simulink model "FL"  (R2017a)
settings: Solver=FixedStepAuto  StartTime=0.0  StopTime=100  FixedStep=0.1  RelTol=1e-3
model workspace: external: MAT-File C:\Users\calvinv\Google Drive\code\Matlab\QuadSim\Simulink\cross_section_model\parameters\param.mat (data not in the file)
settings Model: Creator=calvin  LastModifiedBy=calvinv

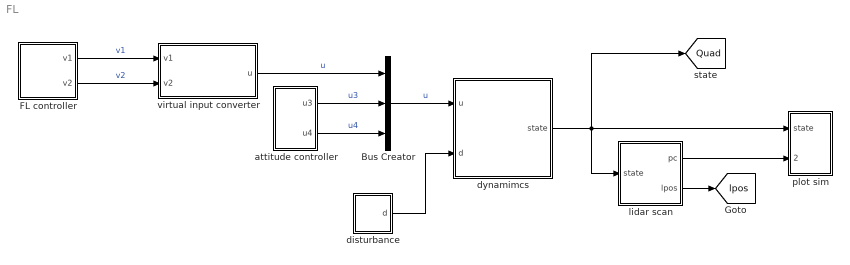
== system FL ==
  Bus Creator : BusCreator  Inputs=3
  FL controller : Subsystem  mask{ky1=10, ky2=42.5, ky3=40.3, ky4=13.4, kz1=10, kz2=42.5, kz3=40.3, kz4=13.4, yd=1, zd=2.5, use_lpos=0}
      mask prompts: yd "target y"; zd "target z"; use_lpos "Use lidar pos feedback"
      mask DialogControl DescGroupVar Prompt: Controller parameters
  attitude controller : Subsystem  mask{P_the=1, D_the=1.5, P_psi=1, D_psi=1.5}
      mask prompts: P_the "Theta P gain"; D_the "Theta D gain"; P_psi "Psi P gain"; D_psi "Pis D gain"
      mask DialogControl DescGroupVar Prompt: Attitude PD controller
  disturbance : Subsystem  mask{freq=20, amp1=0, amp_f=0, amp_tau=0, amp_tau_freq=0, tau_freq=5}
      mask prompts: freq "force oscillation freq"; amp1 "Force amplitude"; amp_f "force oscillation amplitude"; amp_tau "Torque disturbance amplitude"; amp_tau_freq "Torque oscillation freq amp"; tau_freq "Torque oscillation freq"
      mask DialogControl DescGroupVar Prompt: Disturbance generator
  dynamimcs : Subsystem
  lidar scan : Subsystem
  plot sim : Subsystem
  virtual input converter : Subsystem
  tag scope: Quad=global, lpos=global
  wires:
  dynamimcs/1(state) -> lidar scan/1(state), plot sim/1(state), [Quad]
  FL controller/2(v2) -> virtual input converter/2(v2)  "v2"
  FL controller/1(v1) -> virtual input converter/1(v1)  "v1"
  lidar scan/1(pc) -> plot sim/2(lidar pc)
  lidar scan/2(lpos) -> [lpos]
  Bus Creator/1 -> dynamimcs/1(u)  "u"
  attitude controller/1(u3) -> Bus Creator/2  "u3"
  attitude controller/2("u4 ") -> Bus Creator/3  "u4"
  virtual input converter/1(u) -> Bus Creator/1  "u"
  disturbance/1(d) -> dynamimcs/2(d)

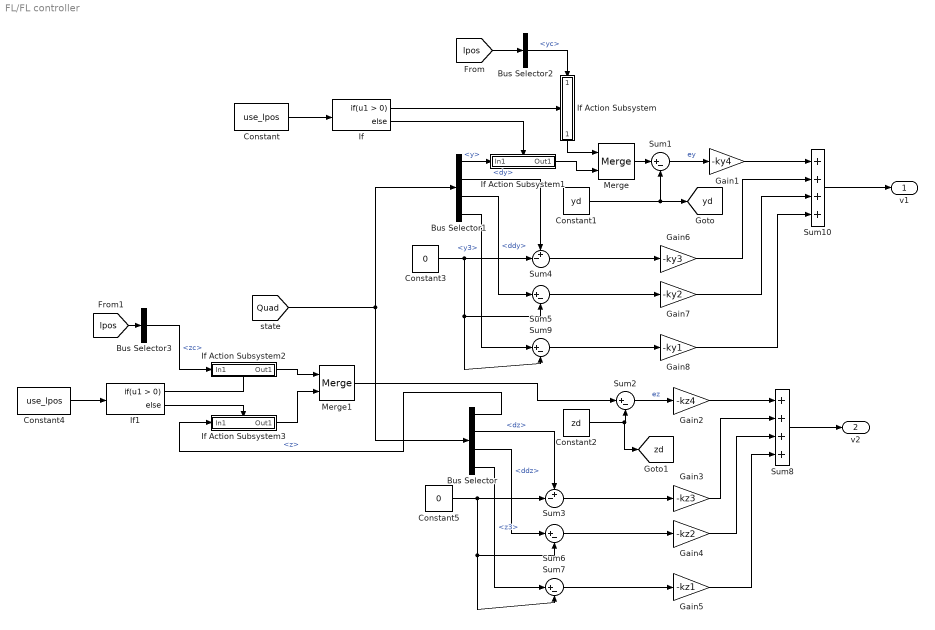
== system FL/FL controller ==
  Bus Selector : BusSelector  OutputSignals=z,dz,ddz,z3
  Bus Selector1 : BusSelector  OutputSignals=y,dy,ddy,y3
  Bus Selector2 : BusSelector  OutputSignals=yc
  Bus Selector3 : BusSelector  OutputSignals=zc
  Constant : Constant  Value=use_lpos
  Constant1 : Constant  Value=yd
  Constant2 : Constant  Value=zd
  Constant3 : Constant  Value=0
  Constant4 : Constant  Value=use_lpos
  Constant5 : Constant  Value=0
  Gain1 : Gain  Gain=-ky4
  Gain2 : Gain  Gain=-kz4
  Gain3 : Gain  Gain=-kz3
  Gain4 : Gain  Gain=-kz2
  Gain5 : Gain  Gain=-kz1
  Gain6 : Gain  Gain=-ky3
  Gain7 : Gain  Gain=-ky2
  Gain8 : Gain  Gain=-ky1
  If : If
  If Action Subsystem : Subsystem  TreatAsAtomicUnit=on
  If Action Subsystem1 : Subsystem  TreatAsAtomicUnit=on
  If Action Subsystem2 : Subsystem  TreatAsAtomicUnit=on
  If Action Subsystem3 : Subsystem  TreatAsAtomicUnit=on
  If1 : If
  Merge : Merge
  Merge1 : Merge
  Sum{1..2,5..7,9} (6 alike) : Sum  Inputs=|+-
  Sum10 : Sum  Inputs=++++
  Sum3 : Sum  Inputs=+-|
  Sum4 : Sum  Inputs=+-|
  Sum8 : Sum  Inputs=++++
  v1 : Outport
  v2 : Outport  Port=2
  tag scope: yd=global, zd=global
  wires:
  Constant5/1 -> Sum7/2, Sum6/2, Sum3/2
  [Quad] -> Bus Selector1/1, Bus Selector/1
  Sum2/1 -> Gain2/1  "ez"
  Constant2/1 -> [zd], Sum2/2
  Bus Selector/2 -> Sum3/1  "<dz>"
  Sum3/1 -> Gain3/1
  Bus Selector/3 -> Sum6/1  "<ddz>"
  Bus Selector/4 -> Sum7/1  "<z3>"
  Sum7/1 -> Gain5/1
  Sum6/1 -> Gain4/1
  Gain2/1 -> Sum8/1
  Sum8/1 -> v2/1
  Gain3/1 -> Sum8/2
  Gain4/1 -> Sum8/3
  Gain5/1 -> Sum8/4
  Gain8/1 -> Sum10/4
  Gain7/1 -> Sum10/3
  Gain6/1 -> Sum10/2
  Sum10/1 -> v1/1
  Gain1/1 -> Sum10/1
  Sum5/1 -> Gain7/1
  Sum9/1 -> Gain8/1
  Bus Selector1/4 -> Sum9/1  "<y3>"
  Bus Selector1/3 -> Sum5/1  "<ddy>"
  Sum4/1 -> Gain6/1
  Bus Selector1/2 -> Sum4/1  "<dy>"
  Constant1/1 -> Sum1/2, [yd]
  Sum1/1 -> Gain1/1  "ey"
  Constant3/1 -> Sum4/2, Sum5/2, Sum9/2
  [lpos] -> Bus Selector2/1
  [lpos] -> Bus Selector3/1
  If/1 -> If Action Subsystem/Action
  If/2 -> If Action Subsystem1/Action
  Bus Selector1/1 -> If Action Subsystem1/1(In1)  "<y>"
  Merge/1 -> Sum1/1
  If Action Subsystem1/1(Out1) -> Merge/2
  If Action Subsystem/1(Out1) -> Merge/1
  Bus Selector2/1 -> If Action Subsystem/1(In1)  "<yc>"
  Constant/1 -> If/1
  If Action Subsystem2/1(Out1) -> Merge1/1
  If Action Subsystem3/1(Out1) -> Merge1/2
  Merge1/1 -> Sum2/1
  If1/1 -> If Action Subsystem2/Action
  If1/2 -> If Action Subsystem3/Action
  Bus Selector3/1 -> If Action Subsystem2/1(In1)  "<zc>"
  Constant4/1 -> If1/1
  Bus Selector/1 -> If Action Subsystem3/1(In1)  "<z>"

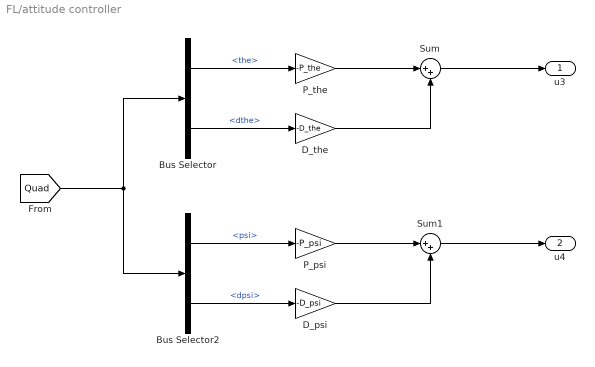
== system FL/attitude controller ==
  Bus Selector : BusSelector  OutputSignals=the,dthe
  Bus Selector2 : BusSelector  OutputSignals=psi,dpsi
  D_psi : Gain  Gain=-D_psi
  D_the : Gain  Gain=-D_the
  P_psi : Gain  Gain=-P_psi
  P_the : Gain  Gain=-P_the
  Sum : Sum  Inputs=|++
  Sum1 : Sum  Inputs=|++
  u3 : Outport
  "u4 " : Outport  Port=2
  wires:
  [Quad] -> Bus Selector2/1, Bus Selector/1
  D_the/1 -> Sum/2
  P_the/1 -> Sum/1
  Bus Selector/2 -> D_the/1  "<dthe>"
  Bus Selector/1 -> P_the/1  "<the>"
  Sum/1 -> u3/1
  Bus Selector2/1 -> P_psi/1  "<psi>"
  Bus Selector2/2 -> D_psi/1  "<dpsi>"
  P_psi/1 -> Sum1/1
  D_psi/1 -> Sum1/2
  Sum1/1 -> "u4 "/1

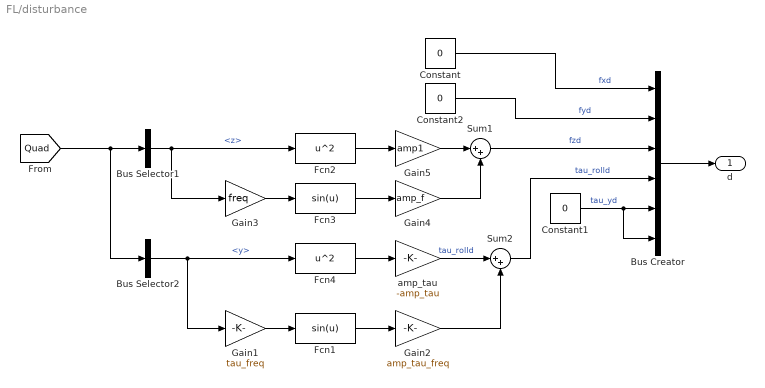
== system FL/disturbance ==
  Bus Creator : BusCreator  Inputs=6
  Bus Selector1 : BusSelector  OutputSignals=z
  Bus Selector2 : BusSelector  OutputSignals=y
  Constant : Constant  Value=0
  Constant1 : Constant  Value=0
  Constant2 : Constant  Value=0
  Fcn1 : Fcn  Expr=sin(u)
  Fcn2 : Fcn  Expr=u^2
  Fcn3 : Fcn  Expr=sin(u)
  Fcn4 : Fcn  Expr=u^2
  Gain1 : Gain  Gain=tau_freq
  Gain2 : Gain  Gain=amp_tau_freq
  Gain3 : Gain  Gain=freq
  Gain4 : Gain  Gain=amp_f
  Gain5 : Gain  Gain=amp1
  Sum1 : Sum  Inputs=|++
  Sum2 : Sum  Inputs=|++
  amp_tau : Gain  Gain=-amp_tau
  d : Outport
  wires:
  [Quad] -> Bus Selector2/1, Bus Selector1/1
  Gain4/1 -> Sum1/2
  Gain5/1 -> Sum1/1
  Bus Selector1/1 -> Fcn2/1, Gain3/1  "<z>"
  Fcn2/1 -> Gain5/1
  Fcn3/1 -> Gain4/1
  Gain3/1 -> Fcn3/1
  Constant2/1 -> Bus Creator/2  "fyd"
  Sum1/1 -> Bus Creator/3  "fzd"
  Constant/1 -> Bus Creator/1  "fxd"
  Bus Creator/1 -> d/1
  Constant1/1 -> Bus Creator/6, Bus Creator/5  "tau_yd"
  Fcn4/1 -> amp_tau/1
  Bus Selector2/1 -> Gain1/1, Fcn4/1  "<y>"
  Gain1/1 -> Fcn1/1
  Fcn1/1 -> Gain2/1
  amp_tau/1 -> Sum2/1  "tau_rolld"
  Gain2/1 -> Sum2/2
  Sum2/1 -> Bus Creator/4  "tau_rolld"

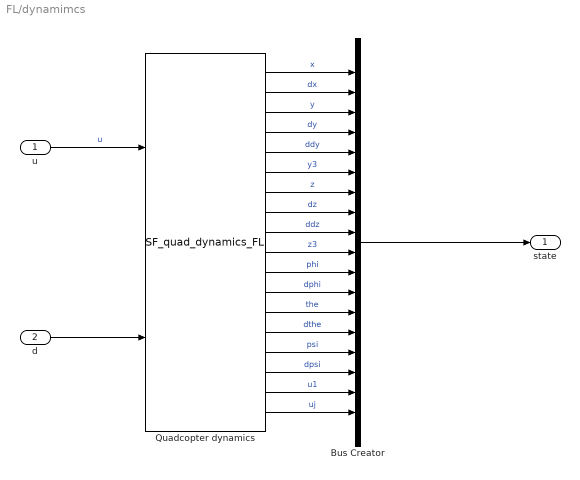
== system FL/dynamimcs ==
  u : Inport
  d : Inport  Port=2
  Bus Creator : BusCreator  Inputs=18
  Quadcopter dynamics : M-S-Function  FunctionName=SF_quad_dynamics_FL  Parameters=quad
  state : Outport
  wires:
  Bus Creator/1 -> state/1
  u/1 -> Quadcopter dynamics/1  "u"
  Quadcopter dynamics/1 -> Bus Creator/1  "x"
  Quadcopter dynamics/2 -> Bus Creator/2  "dx"
  Quadcopter dynamics/3 -> Bus Creator/3  "y"
  Quadcopter dynamics/4 -> Bus Creator/4  "dy"
  Quadcopter dynamics/5 -> Bus Creator/5  "ddy"
  Quadcopter dynamics/6 -> Bus Creator/6  "y3"
  Quadcopter dynamics/7 -> Bus Creator/7  "z"
  Quadcopter dynamics/8 -> Bus Creator/8  "dz"
  Quadcopter dynamics/9 -> Bus Creator/9  "ddz"
  Quadcopter dynamics/10 -> Bus Creator/10  "z3"
  Quadcopter dynamics/11 -> Bus Creator/11  "phi"
  Quadcopter dynamics/12 -> Bus Creator/12  "dphi"
  Quadcopter dynamics/13 -> Bus Creator/13  "the"
  Quadcopter dynamics/14 -> Bus Creator/14  "dthe"
  Quadcopter dynamics/16 -> Bus Creator/16  "dpsi"
  Quadcopter dynamics/17 -> Bus Creator/17  "u1"
  Quadcopter dynamics/15 -> Bus Creator/15  "psi"
  Quadcopter dynamics/18 -> Bus Creator/18  "uj"
  d/1 -> Quadcopter dynamics/2

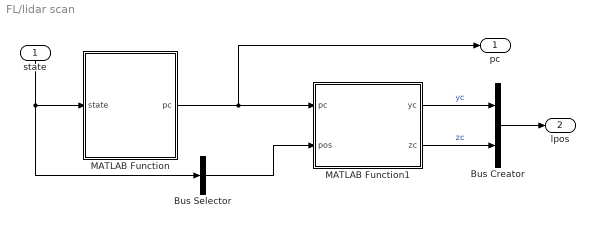
== system FL/lidar scan ==
  state : Inport
  Bus Creator : BusCreator  Inputs=2
  Bus Selector : BusSelector  OutputSignals=y,z  OutputAsBus=on
  MATLAB Function : MATLAB Function  TreatAsAtomicUnit=on
  MATLAB Function1 : MATLAB Function  TreatAsAtomicUnit=on
  pc : Outport
  lpos : Outport  Port=2
  wires:
  state/1 -> MATLAB Function/1(state), Bus Selector/1
  MATLAB Function/1(pc) -> pc/1, MATLAB Function1/1(pc)
  Bus Selector/1 -> MATLAB Function1/2(pos)
  MATLAB Function1/1(yc) -> Bus Creator/1  "yc"
  MATLAB Function1/2(zc) -> Bus Creator/2  "zc"
  Bus Creator/1 -> lpos/1

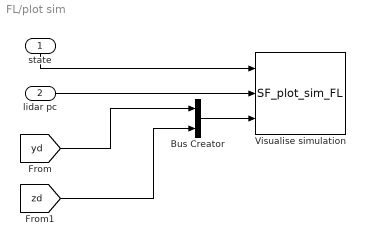
== system FL/plot sim ==
  state : Inport
  lidar pc : Inport  Port=2
  Bus Creator : BusCreator  Inputs=2
  "Visualise simulation " : M-S-Function  FunctionName=SF_plot_sim_FL  Parameters=quad
  wires:
  state/1 -> "Visualise simulation "/1
  lidar pc/1 -> "Visualise simulation "/2
  Bus Creator/1 -> "Visualise simulation "/3
  [yd] -> Bus Creator/1
  [zd] -> Bus Creator/2

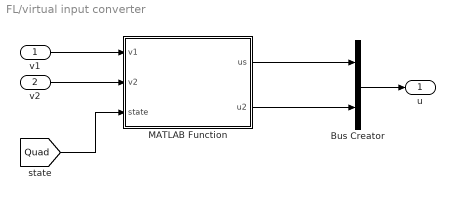
== system FL/virtual input converter ==
  v1 : Inport
  v2 : Inport  Port=2
  Bus Creator : BusCreator  Inputs=2
  MATLAB Function : MATLAB Function  TreatAsAtomicUnit=on
  u : Outport
  wires:
  v2/1 -> MATLAB Function/2(v2)
  [Quad] -> MATLAB Function/3(state)
  MATLAB Function/1(us) -> Bus Creator/1
  MATLAB Function/2(u2) -> Bus Creator/2
  v1/1 -> MATLAB Function/1(v1)
  Bus Creator/1 -> u/1

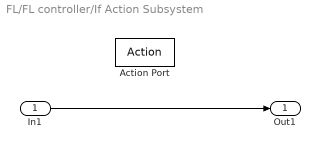
== system FL/FL controller/If Action Subsystem ==
  In1 : Inport
  Action Port : ActionPort  ActionType=then
  Out1 : Outport
  wires:
  In1/1 -> Out1/1

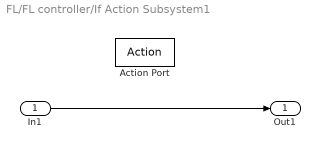
== system FL/FL controller/If Action Subsystem1 ==
  In1 : Inport
  Action Port : ActionPort  ActionType=else
  Out1 : Outport
  wires:
  In1/1 -> Out1/1

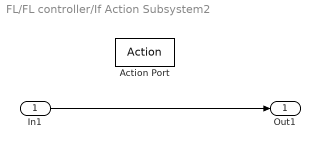
== system FL/FL controller/If Action Subsystem2 ==
  In1 : Inport
  Action Port : ActionPort  ActionType=then
  Out1 : Outport
  wires:
  In1/1 -> Out1/1

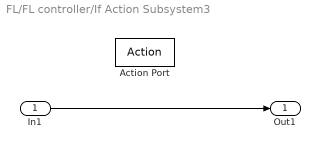
== system FL/FL controller/If Action Subsystem3 ==
  In1 : Inport
  Action Port : ActionPort  ActionType=else
  Out1 : Outport
  wires:
  In1/1 -> Out1/1

== matlab function FL/virtual input converter/MATLAB Function ==
  data: v1 input; us output; v2 input; u2 output; state input
function [us, u2] = v2u(v1, v2, state)

phi = state(11);
dphi = state(12);
u1 = state(17);
uj = state(18);

l = 1;

us = u1 * dphi^2 -sin(phi)*v1 + cos(phi)*v2;

u2 = (-2*dphi*uj - cos(phi)*v1 - sin(phi)*v2)/(l*u1)

== matlab function FL/lidar scan/MATLAB Function ==
  data: state input; pc output
%% need another and condition inside wall check


function pc = lidar_scan_gen(state)

%% init
tunnel_r = 1.5;
tunnel_l = 6; % tunnel length;

a = -135:0.25:135; % lidar FOV is 270 deg

a = a .* pi/180;

pc = zeros(length(a)+5, 3);
temp = zeros(length(a), 3);

z_ceiling = 2 * tunnel_r;
z_ground = 0;

wall_left = -tunnel_r;
wall_right = tunnel_r;

pos_x = state(1);
pos_y = state(3);
pos_z = state(7);
phi = state(11);
the = state(13);
psi = state(15);
the = 0;
psi = 0;

%% checking intersection 
np = 1;
c = 1;
oline = zeros(5,3);

for m = 1:length(a)
    
    angle = [phi the psi];
    
    % generate line point
    r = 20*tunnel_r;
    p = [0 r*sin(a(m)) r*cos(a(m))]';

    pos = [pos_x pos_y pos_z]; % position of the quad
    
    p = Rzyx(angle) * p + pos';    % apply rotation
    
    % wall planes - top right bot left
    n = [0 0 1;0 1 0;0 0 1;0 -1 0];
    wall0 = [0 0 z_ceiling;0 wall_right 0;0 0 z_ground;0 wall_left 0];
    
    for b = 1:4
        [p_wall,check] = plane_line_intersect(n(b, :), wall0(b, :) ,pos ,p');

        if check == 1
            if round(p_wall(2)*1e10)/1e10 > wall_right || round(p_wall(2)*1e10)/1e10 < wall_left
                continue;
            elseif round(p_wall(3)*1e10)/1e10 > z_ceiling || round(p_wall(3)*1e10)/1e10 < z_ground   
                continue;
            else
                break;
            end
        end
    end
    
    % oline is for plotting the centre lines
    
    if m == 1 || m == 1081 || m == 1080/2 || m == 180 || m == 1081-180
        oline(c,:) = p_wall;
        c = c + 1;
    end
    
    lidar_noise = [0 50 - randi(100,1) 50-randi(100,1)]./1000;  % +/- 50mm noise
    
    temp(np,:) = p_wall+ lidar_noise;
    np = np + 1;
end

pc = [oline;temp];

end

== matlab function FL/lidar scan/MATLAB Function1 ==
  data: pc input; yc output; pos input; zc output
function [yc, zc] = get_centroid(pc, pos)

% init
pc = pc(6:end, :);
A = 0;
cy = 0;
cz = 0;

py = pos(1);
pz = pos(2);



y = pc(:,2) + py;
z = pc(:,3) + pz -1.5;

for n = 1:length(pc)-1

    A = A + (y(n) * z(n+1)) - (y(n+1) * z(n));

    cy = cy + (y(n) + y(n+1)) * (y(n) * z(n+1) - y(n+1) * z(n));
    cz = cz + (z(n) + z(n+1)) * (y(n) * z(n+1) - y(n+1) * z(n));
  
end

A = A/2;


pos_loc_y2 = cy/(6 * A);
pos_loc_z2 = cz/(6 * A);



A = -A/(1000^2);
area = A;

yc = pos_loc_y2;
zc = pos_loc_z2;
